simulink model "ADCS2018_Simulink_Full"  (R2018a)
settings: Solver=FixedStepAuto  StartTime=0.0  StopTime=tfinal  FixedStep=ss  RelTol=1e-3  EnableMultiTasking=on
values from neighbouring files (symbols this model uses):
  a1 = -9/11    (= -0.818181818182)    [orbitParameters.m]
  b0 = 2/11    (= 0.181818181818)    [orbitParameters.m]
  b1 = -2/11    (= -0.181818181818)    [orbitParameters.m]
  cr = 1    [orbitParameters.m]
  I = 10^-6*[29290.7 53.8 0.5; 53.8 28639.4 0; 0.5 0 5490.1]    [orbitParameters.m]
  Iw = Hw * 180 / (8000*pi)    [orbitParameters.m]
  Kd = 3.68819*1e-4*0.1/8e-11    (= 461023.75)    [orbitParameters.m]
  kd = 2e-2*min(diag(I))*0.2/3e-9    [orbitParameters.m]
  kep_init = [ semimajoraxis ... (first row only)    [orbitParameters.m]
  Kp = 3.29838*1e-8*0.1/1e-12    (= 3298.38)    [orbitParameters.m]
  mc_max = 0.2    [orbitParameters.m]
  mr = [0.001; -0.001; 0.005]    [orbitParameters.m]
  mr_max = 0.2    [orbitParameters.m]
  omega_o = sqrt(mu/abs(semimajoraxis)^3)    [orbitParameters.m]
  Pitch = 90    [orbitParameters.m]
  Roll = 0    [orbitParameters.m]
  Rx = 30    [orbitParameters.m]
  Ry = 30    [orbitParameters.m]
  Rz = 83    [orbitParameters.m]
  tme_init = [2018 06 07 16 15 0]    [orbitParameters.m]
  vc_max = 5    [orbitParameters.m]
  vr_max = 2.5    [orbitParameters.m]
  wx = 30    [orbitParameters.m]
  wy = 0    [orbitParameters.m]
  wz = 0    [orbitParameters.m]
  Yaw = 0    [orbitParameters.m]
undefined symbols (not defined in the file or in its folder): GHemb, GHsim, sigbuilder_block, SVemb, SVsim, Yemb, Ysim
libraries: My_library x27, simulink x5, vrlib x2, dspindex x1, dspmathops x1
(part 2 of 2)

== matlab function ADCS2018_Simulink_Full/Disturbance/Aerodynamic torque ==
  data: x input; tau_a output; omega_o parameter; kep_init parameter; I parameter
function tau_a   = Adrag(x, omega_o, kep_init, I)
%#codegen

tau_a = zeros(3,1);

m=3.77;
jx = 0.01; %0.05 % X-axis length
jy = 0.01; %0.049 % Y-axis length
jz = 0.03; % Z-axis length
Jx = (m/12)*(jy^2+jz^2); % X-axis inertia
Jy = (m/12)*(jx^2+jz^2); % Y-axis inertia
Jz = (m/12)*(jx^2+jy^2); % Z-axis inertia
J = [Jx 0 0;0 Jy 0;0 0 Jz]; % Inertia matrix

q_B_O = [x(1) ; x(2:4)]';

dcm = zeros(3,3,size(q_B_O,1));
dcm(1,1) = q_B_O(1)^2 + q_B_O(2)^2 - q_B_O(3)^2 - q_B_O(4)^2;
dcm(1,2) = 2*(q_B_O(2)*q_B_O(3) + q_B_O(1)*q_B_O(4));
dcm(1,3) = 2*(q_B_O(2)*q_B_O(4) - q_B_O(1)*q_B_O(3));
dcm(2,1) = 2*(q_B_O(2)*q_B_O(3) - q_B_O(1)*q_B_O(4));
dcm(2,2) = q_B_O(1)^2 - q_B_O(2)^2 + q_B_O(3)^2 - q_B_O(4)^2;
dcm(2,3) = 2*(q_B_O(3)*q_B_O(4) + q_B_O(1)*q_B_O(2));
dcm(3,1) = 2*(q_B_O(2)*q_B_O(4) + q_B_O(1)*q_B_O(3));
dcm(3,2) = 2*(q_B_O(3)*q_B_O(4) - q_B_O(1)*q_B_O(2));
dcm(3,3) = q_B_O(1)^2 - q_B_O(2)^2 - q_B_O(3)^2 + q_B_O(4)^2;

R_B_O = dcm;
w_B_OB =x(5:7);

x = 0.1;
y = 0.1;
z = 0.2;
% A_xo = x*z; % Outer satellite area, x-panel
% A_yo = y*z; % Outer satellite area, y-panel
% A_zo = x*y; % Outer satellite area, z-panel
A_drag = z*sqrt(x^2 + y^2); % Maximum area for calc disturbance drags


vel = kep_init(1)*1e3*omega_o; % Orbit velocity
rho_a = 4.89e-13;

c_p = [0.01 0.01 0.02]';

c_p_x = [0 -c_p(3) c_p(2);
         c_p(3) 0 -c_p(1);
         -c_p(2) c_p(1) 0];

%Vr = R_B_O*[-1 0 0]';

Vr = R_B_O*[0 -1 0]';
Vr_x = [0 -Vr(3) Vr(2);
        Vr(3) 0 -Vr(1);
        -Vr(2) Vr(1) 0];

tau_a = rho_a*vel*( vel*A_drag*c_p_x*Vr-(I + Vr_x*J)*w_B_OB );
tau_a = tau_a(:);

== matlab function ADCS2018_Simulink_Full/Simulation IGRF/IGRFSim ==
  data: P_ECEF input; B_ECEF output; jD input; GHsim parameter; SVsim parameter; Ysim parameter
function B_ECEF = IGRFSim(P_ECEF, jD, GHsim, SVsim, Ysim)


%/ initialisation
B_ECEF=zeros(1,3);


% Fundamental constant.
Rearth_km = 6371.2;


% Convert the latitude, longitude, and altitude coordinates input into
% spherical coordinates r (radius), theta (inclination angle from +z axis),
% and phi (azimuth angle from +x axis).

hypotxy = hypot(P_ECEF(1), P_ECEF(2));
altitude = hypot(hypotxy, P_ECEF(3));
latitude = atan2(P_ECEF(3), hypotxy);
longitude = atan2(P_ECEF(2), P_ECEF(1));

% % We want cos(theta) and sin(theta) rather than theta itself.
costheta = cos(90*pi/180 - latitude);
sintheta = sin(90*pi/180 - latitude);

r = altitude;

phi = longitude;

%%% GET PROPER IGRF COEFFICIENTS %%%
% Convert time to fractional years.
timevec = jD2Dt(jD);
jD = timevec(1) + (jD - Dt2jD([timevec(1) 1 1 0 0 0]))./(365 + double(...
    (~mod(timevec(1),4) & mod(timevec(1),100)) | (~mod(timevec(1),400))));

% Check validity on time.
if jD < Ysim(1) || jD > Ysim(end)
    error('igrf:timeOutOfRange', ['This IGRF is only valid between %d and %d' ...
        Ysim(1) Ysim(end)]);
end

% If one of the coefficient vectors is smaller than the other, enlarge
% the smaller one with 0's.
if length(GHsim) ~= length(SVsim)
    error('igrf:lengthcoefs', 'length(GHsim) ~= length(SVsim)');
end

% Calculate gh using a linear interpolation between the last and next
% epoch.
gh = GHsim + SVsim*(jD - Ysim(1));

nmax = 13;

% We need cos(m*phi) and sin(m*phi) multiple times, so precalculate into a
% vector here:
cosphi = cos((1:nmax)*phi);
sinphi = sin((1:nmax)*phi);

% We need all Legendre polynome, let's first calculate their number
Pmax = (nmax+1)*(nmax+2)/2;

%%% BEGIN MAGNETIC FIELD CALCULATION %%%
% Initialize variables used in for loop below.
Br = 0; Bt = 0; Bp = 0;
 P = zeros(1, Pmax);  P(1) = 1;  P(3) = sintheta;
dP = zeros(1, Pmax); dP(1) = 0; dP(3) = costheta;
% For this initial condition, the first if will result in n = 1, m = 0.
m = 1; n = 0; coefindex = 1;

a_r = (Rearth_km/r)^2;

% Increment through all the n's and m's. gh will be a vector with g
% followed by h for incrementing through n and m except when h would be
% redundant (i.e., when m = 0).
for Pindex = 2:Pmax
    
    % Increment to the next n when m becomes larger than n.
    if n < m
        m = 0;
        n = n + 1;
        a_r = a_r*(Rearth_km/r); % We need (Rearth_km./r)^(n+2)
    end
    
    % Calculate P and dP. They are given recursively according to:
    % 
    % P(0, 0) = 1, P(1, 1) = sin(theta) <- Specified above
    % P(n, n) = sqrt(1 - 1/(2n))*sin(theta)*P(n-1, n-1)
    % P(n, m) = (2n - 1)/sqrt(n^2 - m^2)*cos(theta)*P(n-1, m) -
    %     sqrt(((n-1)^2 - m^2) / (n^2 - m^2)) * P(n-2, m)
    % 
    % dP(0, 0) = 0, dP(1, 1) = cos(theta) <- Specified above
    % dP(n, n) = sqrt(1 - 1/(2n))*(sin(theta)*dP(n-1, n-1) +
    %     cos(theta)*P(n-1, n-1))
    % dP(n, m) = (2n - 1)/sqrt(n^2 - m^2)*(cos(theta)*dP(n-1, m) -
    %     sin(theta)*P(n-1, m)) - sqrt(((n-1)^2 - m^2)/(n^2 - m^2))*
    %     dP(n-2, m)
    if m < n && Pindex ~= 3 % (Pindex=3 is n=1, m=1, initial cond. above)
        last1n = Pindex - n;
        last2n = Pindex - 2*n + 1;
        P(Pindex) = (2*n - 1)/sqrt(n^2 - m^2)*costheta*P(last1n) - ...
            sqrt(((n-1)^2 - m^2) / (n^2 - m^2)) * P(last2n);
        dP(Pindex) = (2*n - 1)/sqrt(n^2 - m^2)*(costheta*dP(last1n) - ...
            sintheta*P(last1n)) - sqrt(((n-1)^2 - m^2) / (n^2 - m^2)) * ...
            dP(last2n);
    elseif Pindex ~= 3
        lastn = Pindex - n - 1;
        P(Pindex) = sqrt(1 - 1/(2*m))*sintheta*P(lastn);
        dP(Pindex) = sqrt(1 - 1/(2*m))*(sintheta*dP(lastn) + ...
            costheta*P(lastn));
    end
    
    % Calculate the magnetic field components as a running sum. Find
    % explicit expressions for these in Global Earth Physics: a Handbook of
    % Physical Constants by Thomas J. Aherns (1995), pg. 49. Link:
    % http://books.google.com/books?id=aqjU_NHyre4C&lpg=PP1&dq=Global%20
    % earth%20physics%3A%20a%20handbook%20of%20physical%20constants&pg=PA49
    % #v=onepage&q&f=false
    % (except equation 6 is missing a required 1/sin(theta) and m; correct
    % equations on page 5 (equations 3a-3c) of:
    % http://hanspeterschaub.info/Papers/UnderGradStudents/
    % MagneticField.pdf)
    if m == 0 % Implies h = 0, so only coefficient in gh is g
        coef = a_r * gh(coefindex); %*cos(0*phi) = 1
        Br = Br + (n+1) .* coef * P(Pindex);
        Bt = Bt - coef * dP(Pindex);
        % Bp is 0 for m = 0.
        coefindex = coefindex + 1; % Only need to skip over g this time.
    else
        coef = a_r * (gh(coefindex) * cosphi(m) + gh(coefindex+1) * sinphi(m));
        Br = Br + (n+1) * coef * P(Pindex);
        Bt = Bt - coef * dP(Pindex);
        if sintheta == 0 % Use different formula when dividing by 0.
            Bp = Bp - costheta*a_r*(-gh(coefindex)*sinphi(m) + ...
                gh(coefindex+1)*cosphi(m))*dP(Pindex);
        else
            Bp = Bp - 1/sintheta*a_r*m*(-gh(coefindex)*sinphi(m) + ...
                gh(coefindex+1)*cosphi(m))*P(Pindex);
        end
        coefindex = coefindex + 2; % Skip over g and h this time.
    end
    
    % Increment m.
    m = m + 1;
    
end
% We need the magnetic field in ECEF coordinate system
coslat=cos(latitude);
sinlat=sin(latitude);
% Convert from spherical to ECEF
Bx = Br*coslat*cosphi(1) + Bt*sinlat*cosphi(1) - Bp*sinphi(1);
By = Br*coslat*sinphi(1) + Bt*sinlat*sinphi(1) - Bp*cosphi(1);
Bz = Br*sinlat - Bt*coslat;

% Convert from nT to T (Tesla)
Bx = Bx * 10^-9;
By = By * 10^-9;
Bz = Bz * 10^-9;

B_ECEF = [Bx, By, Bz];

== matlab function ADCS2018_Simulink_Full/Control/IGRF on bord/IGRFEmb ==
  data: P_ECEF input; B_ECEF output; jD input; GHemb parameter; SVemb parameter; Yemb parameter
function B_ECEF = IGRFEmb(P_ECEF, jD, GHemb, SVemb, Yemb)


%/ initialisation
B_ECEF=zeros(1,3);

% Fundamental constant.
Rearth_km = 6371.2;


% Convert the latitude, longitude, and altitude coordinates input into
% spherical coordinates r (radius), theta (inclination angle from +z axis),
% and phi (azimuth angle from +x axis).

hypotxy = hypot(P_ECEF(1), P_ECEF(2));
altitude = hypot(hypotxy, P_ECEF(3));
latitude = atan2(P_ECEF(3), hypotxy);
longitude = atan2(P_ECEF(2), P_ECEF(1));

% % We want cos(theta) and sin(theta) rather than theta itself.
costheta = cos(90*pi/180 - latitude);
sintheta = sin(90*pi/180 - latitude);

r = altitude;

phi = longitude;

%%% GET PROPER IGRF COEFFICIENTS %%%
% Convert time to fractional years.
timevec = jD2Dt(jD);
jD = timevec(1) + (jD - Dt2jD([timevec(1) 1 1 0 0 0]))./(365 + double(...
    (~mod(timevec(1),4) & mod(timevec(1),100)) | (~mod(timevec(1),400))));

% Check validity on time.
if jD < Yemb(1) || jD > Yemb(end)
    error('igrf:timeOutOfRange', ['This IGRF is only valid between %d and %d' ...
        Yemb(1) Yemb(end)]);
end

% If one of the coefficient vectors is smaller than the other, enlarge
% the smaller one with 0's.
if length(GHemb) ~= length(SVemb)
    error('igrf:lengthcoefs', 'length(GHemb) ~= length(SVemb)');
end

% Calculate gh using a linear interpolation between the last and next
% epoch.
gh = GHemb + SVemb*(jD - Yemb(1));

nmax = 4;

% We need cos(m*phi) and sin(m*phi) multiple times, so precalculate into a
% vector here:
cosphi = cos((1:nmax)*phi);
sinphi = sin((1:nmax)*phi);

% We need all Legendre polynome, let's first calculate their number
Pmax = (nmax+1)*(nmax+2)/2;

%%% BEGIN MAGNETIC FIELD CALCULATION %%%
% Initialize variables used in for loop below.
Br = 0; Bt = 0; Bp = 0;
 P = zeros(1, Pmax);  P(1) = 1;  P(3) = sintheta;
dP = zeros(1, Pmax); dP(1) = 0; dP(3) = costheta;
% For this initial condition, the first if will result in n = 1, m = 0.
m = 1; n = 0; coefindex = 1;

a_r = (Rearth_km/r)^2;

% Increment through all the n's and m's. gh will be a vector with g
% followed by h for incrementing through n and m except when h would be
% redundant (i.e., when m = 0).
for Pindex = 2:Pmax
    
    % Increment to the next n when m becomes larger than n.
    if n < m
        m = 0;
        n = n + 1;
        a_r = a_r*(Rearth_km/r); % We need (Rearth_km./r)^(n+2)
    end
    
    % Calculate P and dP. They are given recursively according to:
    % 
    % P(0, 0) = 1, P(1, 1) = sin(theta) <- Specified above
    % P(n, n) = sqrt(1 - 1/(2n))*sin(theta)*P(n-1, n-1)
    % P(n, m) = (2n - 1)/sqrt(n^2 - m^2)*cos(theta)*P(n-1, m) -
    %     sqrt(((n-1)^2 - m^2) / (n^2 - m^2)) * P(n-2, m)
    % 
    % dP(0, 0) = 0, dP(1, 1) = cos(theta) <- Specified above
    % dP(n, n) = sqrt(1 - 1/(2n))*(sin(theta)*dP(n-1, n-1) +
    %     cos(theta)*P(n-1, n-1))
    % dP(n, m) = (2n - 1)/sqrt(n^2 - m^2)*(cos(theta)*dP(n-1, m) -
    %     sin(theta)*P(n-1, m)) - sqrt(((n-1)^2 - m^2)/(n^2 - m^2))*
    %     dP(n-2, m)
    if m < n && Pindex ~= 3 % (Pindex=3 is n=1, m=1, initial cond. above)
        last1n = Pindex - n;
        last2n = Pindex - 2*n + 1;
        P(Pindex) = (2*n - 1)/sqrt(n^2 - m^2)*costheta*P(last1n) - ...
            sqrt(((n-1)^2 - m^2) / (n^2 - m^2)) * P(last2n);
        dP(Pindex) = (2*n - 1)/sqrt(n^2 - m^2)*(costheta*dP(last1n) - ...
            sintheta*P(last1n)) - sqrt(((n-1)^2 - m^2) / (n^2 - m^2)) * ...
            dP(last2n);
    elseif Pindex ~= 3
        lastn = Pindex - n - 1;
        P(Pindex) = sqrt(1 - 1/(2*m))*sintheta*P(lastn);
        dP(Pindex) = sqrt(1 - 1/(2*m))*(sintheta*dP(lastn) + ...
            costheta*P(lastn));
    end
    
    % Calculate the magnetic field components as a running sum. Find
    % explicit expressions for these in Global Earth Physics: a Handbook of
    % Physical Constants by Thomas J. Aherns (1995), pg. 49. Link:
    % http://books.google.com/books?id=aqjU_NHyre4C&lpg=PP1&dq=Global%20
    % earth%20physics%3A%20a%20handbook%20of%20physical%20constants&pg=PA49
    % #v=onepage&q&f=false
    % (except equation 6 is missing a required 1/sin(theta) and m; correct
    % equations on page 5 (equations 3a-3c) of:
    % http://hanspeterschaub.info/Papers/UnderGradStudents/
    % MagneticField.pdf)
    if m == 0 % Implies h = 0, so only coefficient in gh is g
        coef = a_r * gh(coefindex); %*cos(0*phi) = 1
        Br = Br + (n+1) .* coef * P(Pindex);
        Bt = Bt - coef * dP(Pindex);
        % Bp is 0 for m = 0.
        coefindex = coefindex + 1; % Only need to skip over g this time.
    else
        coef = a_r * (gh(coefindex) * cosphi(m) + gh(coefindex+1) * sinphi(m));
        Br = Br + (n+1) * coef * P(Pindex);
        Bt = Bt - coef * dP(Pindex);
        if sintheta == 0 % Use different formula when dividing by 0.
            Bp = Bp - costheta*a_r*(-gh(coefindex)*sinphi(m) + ...
                gh(coefindex+1)*cosphi(m))*dP(Pindex);
        else
            Bp = Bp - 1/sintheta*a_r*m*(-gh(coefindex)*sinphi(m) + ...
                gh(coefindex+1)*cosphi(m))*P(Pindex);
        end
        coefindex = coefindex + 2; % Skip over g and h this time.
    end
    
    % Increment m.
    m = m + 1;
    
end
% We need the magnetic field in ECEF coordinate system
coslat=cos(latitude);
sinlat=sin(latitude);
% Convert from spherical to ECEF
Bx = Br*coslat*cosphi(1) + Bt*sinlat*cosphi(1) - Bp*sinphi(1);
By = Br*coslat*sinphi(1) + Bt*sinlat*sinphi(1) - Bp*cosphi(1);
Bz = Br*sinlat - Bt*coslat;

% Convert from nT to T (Tesla)
Bx = Bx * 10^-9;
By = By * 10^-9;
Bz = Bz * 10^-9;

B_ECEF = [Bx, By, Bz];

== matlab function ADCS2018_Simulink_Full/X_bi 2 X_bo /Propagator ==
  settings: sampleTime=1
  data: V_TEME output; t input; P_TEME output; kep_init parameter; Q_oi output; W_oi_o output
function [V_TEME, P_TEME, Q_oi, W_oi_o]  = pos(t, kep_init)
%#codegen

coder.extrinsic('PVOrb')

P_TEME = zeros(3,1);
V_TEME = zeros(3,1);
W_oi_o = zeros(3,1);

[P_TEME,V_TEME] = PVOrb(kep_init,t);
P_TEME = P_TEME(:);
V_TEME = V_TEME(:);

NormP2 = P_TEME(1) * P_TEME(1) + P_TEME(2) * P_TEME(2) + P_TEME(3) * P_TEME(3);
W_oi_o = cross(V_TEME, P_TEME) / NormP2;

Q_oi = Qorb(P_TEME, V_TEME);

end

== matlab function ADCS2018_Simulink_Full/X_bo  2  X_bi/Propagator1 ==
  settings: sampleTime=1
  data: V_TEME output; t input; P_TEME output; kep_init parameter; Q_oi output; W_oi_o output
function [V_TEME, P_TEME, Q_oi, W_oi_o]  = pos(t, kep_init)
%#codegen

coder.extrinsic('PVOrb')

P_TEME = zeros(3,1);
V_TEME = zeros(3,1);
W_oi_o = zeros(3,1);

[P_TEME,V_TEME] = PVOrb(kep_init,t);
P_TEME = P_TEME(:);
V_TEME = V_TEME(:);

NormP2 = P_TEME(1) * P_TEME(1) + P_TEME(2) * P_TEME(2) + P_TEME(3) * P_TEME(3);
W_oi_o = cross(V_TEME, P_TEME) / NormP2;

Q_oi = Qorb(P_TEME, V_TEME);

end

== matlab function ADCS2018_Simulink_Full/Simulation IGRF/Propagator ==
  settings: sampleTime=1
  data: V_TEME output; t input; P_TEME output; kep_init parameter
function [V_TEME, P_TEME]  = pos(t, kep_init)
%#codegen

coder.extrinsic('PVOrb')
P_TEME=zeros(3,1);
V_TEME=zeros(3,1);

[P_TEME,V_TEME] = PVOrb(kep_init,t);
P_TEME=P_TEME(:);
V_TEME=V_TEME(:);


end

== matlab function ADCS2018_Simulink_Full/Simulation IGRF/MATLAB Function1 ==
  data: t input; T_JD output; tme_init parameter
function T_JD = fcn(t, tme_init)
%#codegen
tme_init(6)=tme_init(6)+t;
T_JD=Dt2jD(tme_init);

== matlab function ADCS2018_Simulink_Full/Control/IGRF on bord/Propagator ==
  settings: sampleTime=1
  data: V_TEME output; t input; P_TEME output; Q_oi output; kep_init input
function [V_TEME, P_TEME, Q_oi]  = pos(t, kep_init)
%#codegen

coder.extrinsic('PVOrb')
P_TEME=zeros(3,1);
V_TEME=zeros(3,1);

[P_TEME,V_TEME] = PVOrb(kep_init,t);
P_TEME=P_TEME(:);
V_TEME=V_TEME(:);


Q_oi=Qorb(P_TEME, V_TEME);

end
